simulink subsystem "VehicleBody3DOFLongitudinalSSC"  (R2025a)
settings: Solver=VariableStepAuto  StartTime=0.0  StopTime=10.0  RelTol=1e-3
undefined symbols (not defined in the file): EnvGrvty, PlntVeh3DOFFrntSuspStiff, PlntVeh3DOFRearSuspStiff, PlntVehCGHgtAxl, PlntVehDstCGFrntAxl, PlntVehDstCGRearAxl, PlntVehHtchDst, PlntVehHtchHgtAxl, PlntVehHtchLatDst, PlntWhlLdRadiusFrnt
libraries: nesl_utility_internal x5, nesl_utility x4, fl_lib x3, sdl_lib x1
settings Model: ModifiedByFormat=The MathWorks, Inc.  Creator=The MathWorks, Inc.  LastModifiedBy=The MathWorks, Inc.
settings OptimizationCC: ReuseModelBlockBuffer=off
settings DebuggingCC: SubsystemReferenceDiagnosticForUnitTest=warning
settings RTWCC: GPUComputeCapability=3.5

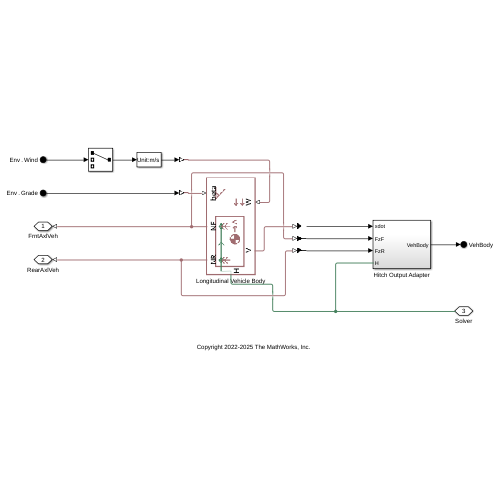
[thumbnail: Simulink's stored preview of the top-level diagram]
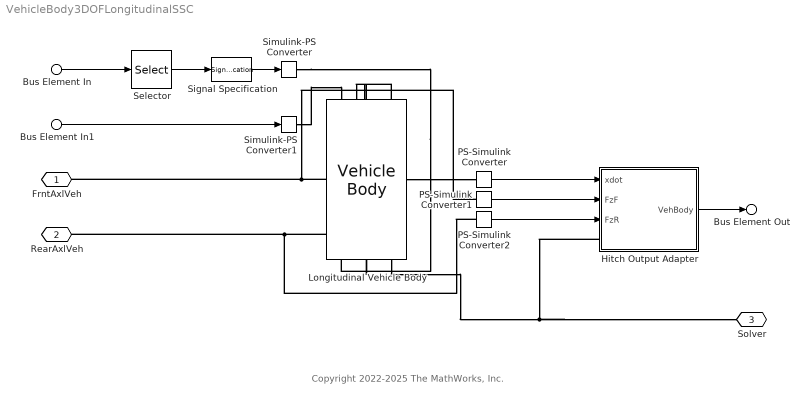
== system VehicleBody3DOFLongitudinalSSC ==
  note: Copyright 2022-2025 The MathWorks, Inc.
  Bus Element In : Inport  PortName=Env  Element=Wind
  Bus Element In1 : Inport  PortName=Env  Element=Grade
  Hitch Output Adapter : Subsystem
  Longitudinal Vehicle Body : sdl_lib/Tires & Vehicles/Vehicle Body  mass=PlntVehMass kg  n_w=PlntVehNumWhlFrntAxl  x_f=PlntVehDstCGFrntAxl m  x_r=PlntVehDstCGRearAxl m  y_c=PlntVehCGHgtAxl+PlntWhlLdRadiusFrnt m  mass_var=simscape.enum.onoff.off  g=EnvGrvty m/s^2  liftoff_warning=simscape.enum.onoff.off  area=PlntVehAeroFrntArea m^2  Cd_var=false  Cd=PlntVehAeroDragCff  rho=EnvAirDen kg/m^3  model_pitch=simscape.enum.onoff.on  inertia=PlntVehPitchMomentInertia kg*m^2  suspension_model=sdl.enum.linearTLU.linear  k_f=PlntVeh3DOFFrntSuspStiff N/m  b_f=PlntVeh3DOFFrntSuspDamp N*s/m  k_r=PlntVeh3DOFRearSuspStiff N/m  b_r=PlntVeh3DOFRearSuspDamp N*s/m  k_f_TLU=[-2000, -1000, 0, 1000, 2000] N  x_f_TLU=[-.4, -.2, 0, .2, .4] m  b_f_TLU=[-200, -100, 0, 100, 200] N  v_f_TLU=[-4, -2, 0, 2, 4] m/s  k_r_TLU=[-2000, -1000, 0, 1000, 2000] N  x_r_TLU=[-.4, -.2, 0, .2, .4] m  b_r_TLU=[-200, -100, 0, 100, 200] N  v_r_TLU=[-4, -2, 0, 2, 4] m/s  interp_method=simscape.enum.interpolation.linear  extrap_method=simscape.enum.extrapolation.linear  model_hardstop=simscape.enum.onoff.off  upper_bound_f=.25 m  lower_bound_f=-.25 m  stop_k_f=1e6 N/m  stop_b_f=150 N*s/m  upper_bound_r=.25 m  lower_bound_r=-.25 m  stop_k_r=1e6 N/m  stop_b_r=150 N*s/m  initial_pitch=PlntVehInitPitchAng rad  initial_pitch_rate=PlntVehInitPitchRate rad/s  v_specify=off  v_priority=High  v=0 m/s  v_nominal_specify=off  v_nominal_value=1  v_nominal_unit=m/s
      settings: InternalSimscapePortConfiguration="{\"Bottom\":[{\"id\":\"NR\",\"label\":\"NR\",\"type\":\"output\"},{\"id\":\"NF\",\"label\":\"NF\",\"type\":\"output\"},{\"id\":\"beta\",\"label\":\"beta\",\"type\":\"input\"}],\"Left\":[{\"id\":\"H\",\"label\":\"H\",\"type\":\"foundation.mechanical.translational.translational\"}],\"Right\":[],\"Top\":[{\"id\":\"V\",\"label\":\"V\",\"type\":\"output\"},{\"id\":\"wind\",\"label\":\"W\",\"type\":\"input\"}]}"
  PS-Simulink Converter : nesl_utility_internal/PS-Simulink Converter  PhysicalDomain=network_engine_domain  SubClassName=ps_output  LeftPortType=input  RightPortType=output  PseudoPeriodic=off  Frequencies=[]  VectorFormat=inherit  Unit=inherit  AffineConversion=off
  PS-Simulink Converter1 : nesl_utility_internal/PS-Simulink Converter  PhysicalDomain=network_engine_domain  SubClassName=ps_output  LeftPortType=input  RightPortType=output  PseudoPeriodic=off  Frequencies=[]  VectorFormat=inherit  Unit=inherit  AffineConversion=off
  PS-Simulink Converter2 : nesl_utility_internal/PS-Simulink Converter  PhysicalDomain=network_engine_domain  SubClassName=ps_output  LeftPortType=input  RightPortType=output  PseudoPeriodic=off  Frequencies=[]  VectorFormat=inherit  Unit=inherit  AffineConversion=off
  Selector : Selector  InputPortWidth=3  IndexOptions=Index vector (dialog)  Indices=[1]  OutputSizes=1
  Signal Specification : SignalSpecification  Unit=m/s
  Simulink-PS Converter : nesl_utility_internal/Simulink-PS Converter  PhysicalDomain=network_engine_domain  SubClassName=ps_input  LeftPortType=input  RightPortType=output  PseudoPeriodic=off  Frequencies=[]  NoiseDistribution=none  NoiseParameters=[]  Unit=m/s  AffineConversion=off  FilteringAndDerivatives=provide  SimscapeFilterOrder=1  InputFilterTimeConstant=0.001  UdotUserProvided=0
  Simulink-PS Converter1 : nesl_utility_internal/Simulink-PS Converter  PhysicalDomain=network_engine_domain  SubClassName=ps_input  LeftPortType=input  RightPortType=output  PseudoPeriodic=off  Frequencies=[]  NoiseDistribution=none  NoiseParameters=[]  Unit=deg  AffineConversion=off  FilteringAndDerivatives=provide  SimscapeFilterOrder=1  InputFilterTimeConstant=0.001  UdotUserProvided=0
  FrntAxlVeh : PMIOPort  Side=Left
  RearAxlVeh : PMIOPort  Port=2  Side=Left
  Solver : PMIOPort  Port=3  Side=Right
  Bus Element Out : Outport  PortName=VehBody
  wires:
  Hitch Output Adapter/1(VehBody) -> Bus Element Out/1
  Signal Specification/1 -> Simulink-PS Converter/1
  PS-Simulink Converter/1 -> Hitch Output Adapter/1(xdot)
  PS-Simulink Converter1/1 -> Hitch Output Adapter/2(FzF)
  Selector/1 -> Signal Specification/1
  PS-Simulink Converter2/1 -> Hitch Output Adapter/3(FzR)
  Bus Element In1/1 -> Simulink-PS Converter1/1
  Bus Element In/1 -> Selector/1
  connections:
  PS-Simulink Converter2/LConn1 -- RearAxlVeh/RConn1 -- Longitudinal Vehicle Body/RConn1
  PS-Simulink Converter1/LConn1 -- FrntAxlVeh/RConn1 -- Longitudinal Vehicle Body/RConn2
  Hitch Output Adapter/LConn1 -- Longitudinal Vehicle Body/LConn1 -- Solver/RConn1
  Longitudinal Vehicle Body/LConn2 -- PS-Simulink Converter/LConn1
  Simulink-PS Converter1/RConn1 -- Longitudinal Vehicle Body/RConn3
  Simulink-PS Converter/RConn1 -- Longitudinal Vehicle Body/LConn3

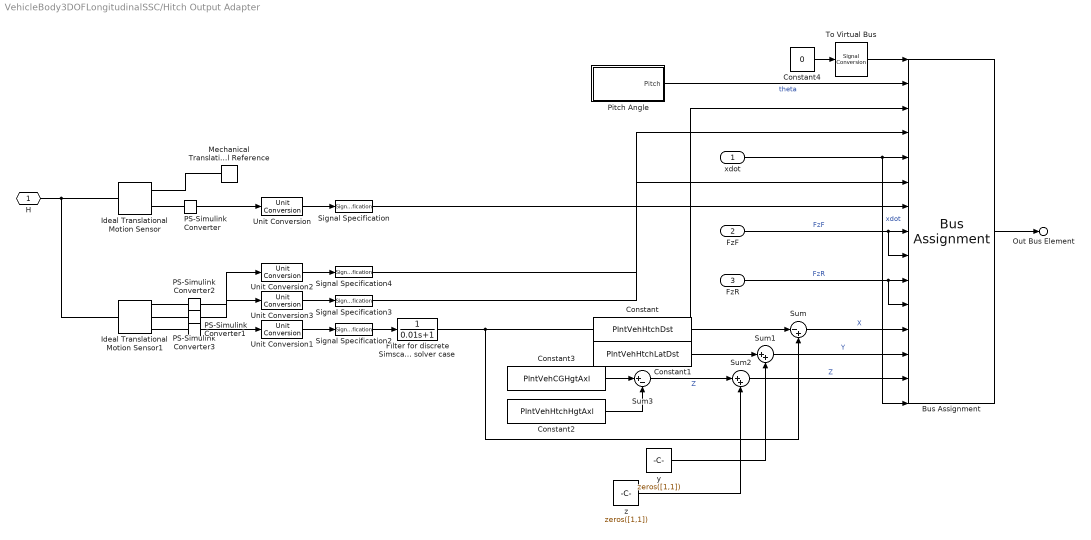
== system VehicleBody3DOFLongitudinalSSC/Hitch Output Adapter ==
  xdot : Inport
  FzF : Inport  Port=2
  FzR : Inport  Port=3
  Bus Assignment : BusAssignment  AssignedSignals=InertFrm.Cg.Ang.theta,InertFrm.Cg.Disp.X,InertFrm.Cg.Vel.Xdot,BdyFrm.Cg.Vel.xdot,BdyFrm.Cg.Acc.xddot,BdyFrm.Cg.Acc.ax,BdyFrm.Forces.FrntAxl.Lft.Fz,BdyFrm.Forces.FrntAxl.Rght.Fz,BdyFrm.Forces.RearAxl.Lft.Fz,BdyFrm.Forces.RearAxl.Rght.Fz,InertFrm.Hitch.Disp.X,InertFrm.Hitch.Disp.Y,InertFrm.Hitch.Disp.Z,InertFrm.Hitch.Vel.Xdot
  Constant : Constant  Value=PlntVehHtchDst  SampleTime=-1
  Constant1 : Constant  Value=PlntVehHtchLatDst  SampleTime=-1
  Constant2 : Constant  Value=PlntVehHtchHgtAxl  SampleTime=-1
  Constant3 : Constant  Value=PlntVehCGHgtAxl  SampleTime=-1
  Constant4 : Constant  Value=0  OutDataTypeStr=Bus: VehBodyBUS  SampleTime=Inf
  Filter for discrete Simscape solver case : TransferFcn  Denominator=[0.01 1]
  Ideal Translational Motion Sensor : fl_lib/Mechanical/Mechanical Sensors/Ideal Translational Motion Sensor  reference=foundation.enum.MeasurementReference.difference  acceleration_port=true  velocity_port=false  position_port=false  offset=0 m
      settings: InternalSimscapePortConfiguration="{\"Bottom\":[],\"Left\":[{\"id\":\"R\",\"label\":\"R\",\"type\":\"foundation.mechanical.translational.translational\"}],\"Right\":[{\"id\":\"C\",\"label\":\"C\",\"type\":\"foundation.mechanical.translational.translational\"},{\"id\":\"A\",\"label\":\"A\",\"type\":\"output\"}],\"Top\":[]}"
  Ideal Translational Motion Sensor1 : fl_lib/Mechanical/Mechanical Sensors/Ideal Translational Motion Sensor  reference=foundation.enum.MeasurementReference.absolute  acceleration_port=true  velocity_port=true  position_port=true  offset=0 m
      settings: InternalSimscapePortConfiguration="{\"Bottom\":[],\"Left\":[{\"id\":\"R\",\"label\":\"R\",\"type\":\"foundation.mechanical.translational.translational\"}],\"Right\":[{\"id\":\"A\",\"label\":\"A\",\"type\":\"output\"},{\"id\":\"V\",\"label\":\"V\",\"type\":\"output\"},{\"id\":\"P\",\"label\":\"P\",\"type\":\"output\"}],\"Top\":[]}"
  Mechanical Translational Reference : fl_lib/Mechanical/Translational Elements/Mechanical Translational Reference
  PS-Simulink Converter{,1..3} (4 alike) : nesl_utility/PS-Simulink Converter  PhysicalDomain=network_engine_domain  SubClassName=ps_output  LeftPortType=input  RightPortType=output  PseudoPeriodic=off  Frequencies=[]  VectorFormat=inherit  Unit=inherit  AffineConversion=off
  Pitch Angle : Subsystem
  Signal Specification : SignalSpecification  Unit=gn
  Signal Specification2 : SignalSpecification  Unit=m
  Signal Specification3 : SignalSpecification  Unit=m/s
  Signal Specification4 : SignalSpecification  Unit=m/s^2
  Sum : Sum  Inputs=|-+
  Sum1 : Sum  Inputs=|++
  Sum2 : Sum  Inputs=|++
  Sum3 : Sum  Inputs=|+-
  To Virtual Bus : SignalConversion  ConversionOutput=Virtual bus  OverrideOpt=off
  Unit Conversion{,1..3} (4 alike) : UnitConversion
  y : Constant  Value=zeros([1,1])  SampleTime=-1
  z : Constant  Value=zeros([1,1])  SampleTime=-1
  H : PMIOPort  Side=Left
  Out Bus Element : Outport  PortName=VehBody
  wires:
  Pitch Angle/1(Pitch) -> Bus Assignment/2  "theta"
  Unit Conversion/1 -> Signal Specification/1
  PS-Simulink Converter/1 -> Unit Conversion/1
  To Virtual Bus/1 -> Bus Assignment/1
  Bus Assignment/1 -> Out Bus Element/1
  Constant4/1 -> To Virtual Bus/1
  z/1 -> Sum2/2
  Signal Specification2/1 -> Filter for discrete Simscape solver case/1
  y/1 -> Sum1/2
  Constant/1 -> Sum/1
  Sum3/1 -> Sum2/1  "Z"
  Constant3/1 -> Sum3/1
  Sum2/1 -> Bus Assignment/14  "Z"
  Constant2/1 -> Sum3/2
  Sum/1 -> Bus Assignment/12  "X"
  Sum1/1 -> Bus Assignment/13  "Y"
  Constant1/1 -> Sum1/1
  Unit Conversion2/1 -> Signal Specification4/1
  Unit Conversion1/1 -> Signal Specification2/1
  PS-Simulink Converter2/1 -> Unit Conversion2/1
  PS-Simulink Converter3/1 -> Unit Conversion3/1
  PS-Simulink Converter1/1 -> Unit Conversion1/1
  Unit Conversion3/1 -> Signal Specification3/1
  Signal Specification/1 -> Bus Assignment/7
  Signal Specification4/1 -> Bus Assignment/6
  Signal Specification3/1 -> Bus Assignment/4
  Filter for discrete Simscape solver case/1 -> Bus Assignment/3, Sum/2
  xdot/1 -> Bus Assignment/5, Bus Assignment/15  "xdot"
  FzF/1 -> Bus Assignment/8, Bus Assignment/9  "FzF"
  FzR/1 -> Bus Assignment/10, Bus Assignment/11  "FzR"
  connections:
  Mechanical Translational Reference/LConn1 -- Ideal Translational Motion Sensor/RConn1
  PS-Simulink Converter/LConn1 -- Ideal Translational Motion Sensor/RConn2
  H/RConn1 -- Ideal Translational Motion Sensor/LConn1 -- Ideal Translational Motion Sensor1/LConn1
  Ideal Translational Motion Sensor1/RConn3 -- PS-Simulink Converter1/LConn1
  Ideal Translational Motion Sensor1/RConn1 -- PS-Simulink Converter2/LConn1
  Ideal Translational Motion Sensor1/RConn2 -- PS-Simulink Converter3/LConn1

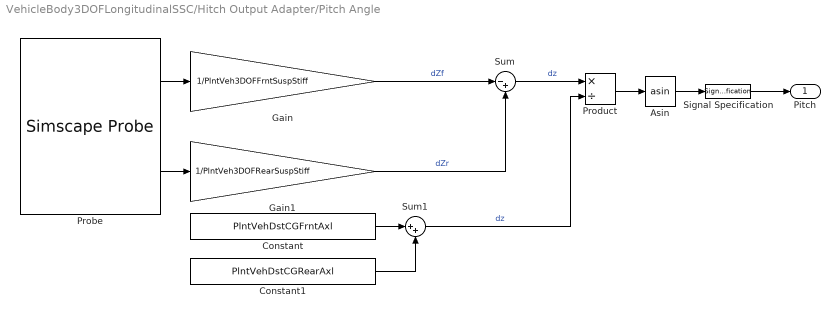
== system VehicleBody3DOFLongitudinalSSC/Hitch Output Adapter/Pitch Angle ==
  Asin : Trigonometry  Operator=asin
  Constant : Constant  Value=PlntVehDstCGFrntAxl
  Constant1 : Constant  Value=PlntVehDstCGRearAxl
  Gain : Gain  Gain=1/PlntVeh3DOFFrntSuspStiff
  Gain1 : Gain  Gain=1/PlntVeh3DOFRearSuspStiff
  Probe : SimscapeProbe  BoundBlock=24445  Variables="{\"suspension_force_f\":{\"Probing\":\"ON\"},\"suspension_force_r\":{\"Probing\":\"ON\"}}"
  Product : Product  Inputs=*/
  Signal Specification : SignalSpecification  Unit=rad
  Sum : Sum  Inputs=|-+
  Sum1 : Sum  Inputs=|++
  Pitch : Outport
  wires:
  Signal Specification/1 -> Pitch/1
  Constant/1 -> Sum1/1
  Asin/1 -> Signal Specification/1
  Sum1/1 -> Product/2  "dz"
  Constant1/1 -> Sum1/2
  Sum/1 -> Product/1  "dz"
  Gain1/1 -> Sum/2  "dZr"
  Gain/1 -> Sum/1  "dZf"
  Product/1 -> Asin/1
  Probe/2 -> Gain1/1
  Probe/1 -> Gain/1
